simulink model "BSC"  (R2015b)
settings: Solver=FixedStepDiscrete  StartTime=0.0  StopTime=inf  FixedStep=bsck_stepSize  RelTol=1e-3
PreLoadFcn:
  | openecu_make_rtw_hook('model_load',   'BSC')
PostLoadFcn:
  | openecu_make_rtw_hook('model_loaded', 'BSC')
InitFcn:
  | openecu_make_rtw_hook('model_init',   'BSC')
undefined symbols (not defined in the file or in its folder): bscv_LowFaultType, bscv_MediumFaultType, bscv_SevereFaultType
libraries: simulink x4
settings Model: Creator=nctzv8  LastModifiedBy=nctzv8
settings ConfigSet: Description=OpenECU configuration set for code generation under RTW-EC.
settings SolverCC: PositivePriorityOrder=on
settings DataIOCC: SaveFormat=Array  SignalLoggingSaveFormat=ModelDataLogs
settings OptimizationCC: DefaultParameterBehavior=Inlined  InlineInvariantSignals=on  ExpressionDepthLimit=2147483647  StateBitsets=on  DataBitsets=on  ZeroExternalMemoryAtStartup=off  ZeroInternalMemoryAtStartup=off  NoFixptDivByZeroProtection=on  EfficientFloat2IntCast=on  OptimizeModelRefInitCode=on  LifeSpan=1
settings DebuggingCC: SaveWithParameterizedLinksMsg=none  UnderspecifiedInitializationDetection=Classic  MergeDetectMultiDrivingBlocksExec=none  SignalResolutionControl=TryResolveAllWithWarning  MultiTaskDSMMsg=warning  MultiTaskCondExecSysMsg=none  SingleTaskRateTransMsg=error  CheckMatrixSingularityMsg=warning  VectorMatrixConversionMsg=warning  FcnCallInpInsideContextMsg=UseLocalSettings  SignalLabelMismatchMsg=warning  StateNameClashWarn=warning
settings HardwareCC: ProdBitPerPointer=32  ProdLargestAtomicInteger=Long  ProdLargestAtomicFloat=Double  ProdEndianess=BigEndian  ProdWordSize=32  ProdHWDeviceType=Freescale->32-bit PowerPC  TargetIntDivRoundTo=Zero  TargetEndianess=BigEndian  TargetHWDeviceType=Freescale->32-bit PowerPC  ProdEqTarget=off
settings RTWCC: SystemTargetFile=openecu_ert.tlc  MakeCommand=make_rtw optimized_floating_point=1  TemplateMakefile=openecu_ert_r2015b_64.tmf  Description=OpenECU Platform Target (ERT, optimised floating-point code)  GenerateReport=on  RetainRTWFile=on  IncludeHyperlinkInReport=on  LaunchReport=on
settings CodeAppCC: ForceParamTrailComments=on  IgnoreCustomStorageClasses=off  SimulinkDataObjDesc=on  CustomSymbolStrType=$N$R$M  InsertBlockDesc=on  InternalIdentifier=Classic
settings STFCustomTargetCC: TargetLibSuffix=.a  GenerateSampleERTMain=on  ConcurrentExecutionCompliant=off  IncludeMdlTerminateFcn=off  GeneratePreprocessorConditionals=Use local settings  CombineOutputUpdateFcns=on  IncludeFileDelimiter=UseQuote  ERTCustomFileBanners=on  SupportContinuousTime=off  MATLABClassNameForMDSCustomization=Simulink.SoftwareTarget.ERTCustomization  CPPClassGenCompliant=off  GRTInterface=off  SystemTargetFile=openecu_ert.tlc
settings ERTTargetCC: GenerateSampleERTMain=on  ParMdlRefBuildCompliant=off  CompOptLevelCompliant=off  ConcurrentExecutionCompliant=off  IncludeMdlTerminateFcn=off  ERTFirstTimeCompliant=off  IncludeFileDelimiter=UseQuote  SupportNonInlinedSFcns=on  ModelStepFunctionPrototypeControlCompliant=off  CPPClassGenCompliant=off  UseToolchainInfoCompliant=off  ExtModeMexFile=noextcomm  InlinedParameterPlacement=NonHierarchical  ERTSrcFileBannerTemplate=oe_code_c_template.cgt  ERTHdrFileBannerTemplate=oe_code_h_template.cgt  ERTDataSrcFileTemplate=oe_data_c_template.cgt  ERTDataHdrFileTemplate=oe_data_h_template.cgt  ERTCustomFileTemplate=example_file_process.tlc  GlobalDataDefinition=InSeparateSourceFile  GlobalDataReference=InSeparateHeaderFile  EnableUserReplacementTypes=on

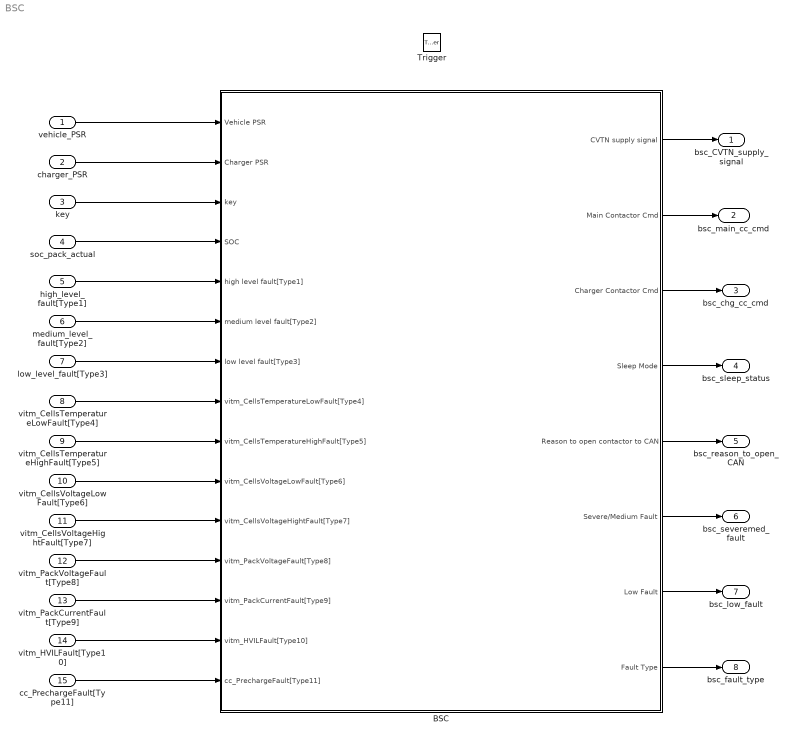
== system BSC ==
  vehicle_PSR : Inport  OutDataTypeStr=uint8  PortDimensions=1
  charger_PSR : Inport  Port=2  OutDataTypeStr=uint8  PortDimensions=1
  key : Inport  Port=3  OutDataTypeStr=uint8  PortDimensions=1
  soc_pack_actual : Inport  Port=4  OutDataTypeStr=double  PortDimensions=1
  high_level_fault[Type1] : Inport  Port=5  OutDataTypeStr=uint8  PortDimensions=1
  medium_level_fault[Type2] : Inport  Port=6  OutDataTypeStr=uint8  PortDimensions=1
  low_level_fault[Type3] : Inport  Port=7  OutDataTypeStr=uint8  PortDimensions=1
  vitm_CellsTemperatureLowFault[Type4] : Inport  Port=8  OutDataTypeStr=uint8  PortDimensions=1
  vitm_CellsTemperatureHighFault[Type5] : Inport  Port=9  OutDataTypeStr=uint8  PortDimensions=1
  vitm_CellsVoltageLowFault[Type6] : Inport  Port=10  OutDataTypeStr=uint8  PortDimensions=1
  vitm_CellsVoltageHightFault[Type7] : Inport  Port=11  OutDataTypeStr=uint8  PortDimensions=1
  vitm_PackVoltageFault[Type8] : Inport  Port=12  OutDataTypeStr=uint8  PortDimensions=1
  vitm_PackCurrentFault[Type9] : Inport  Port=13  OutDataTypeStr=uint8  PortDimensions=1
  vitm_HVILFault[Type10] : Inport  Port=14  OutDataTypeStr=uint8  PortDimensions=1
  cc_PrechargeFault[Type11] : Inport  Port=15  OutDataTypeStr=uint8  PortDimensions=1
  Trigger : TriggerPort  TriggerType=function-call  PortDimensions=1
  BSC : Subsystem  TreatAsAtomicUnit=on
  bsc_CVTN_supply_signal : Outport  OutDataTypeStr=boolean  PortDimensions=1
  bsc_main_cc_cmd : Outport  Port=2  OutDataTypeStr=boolean  PortDimensions=1
  bsc_chg_cc_cmd : Outport  Port=3  OutDataTypeStr=boolean  PortDimensions=1
  bsc_sleep_status : Outport  Port=4  OutDataTypeStr=boolean  PortDimensions=1
  bsc_reason_to_open_CAN : Outport  Port=5  OutDataTypeStr=uint8  PortDimensions=1
  bsc_severemed_fault : Outport  Port=6  OutDataTypeStr=uint8  PortDimensions=1
  bsc_low_fault : Outport  Port=7  OutDataTypeStr=uint8  PortDimensions=1
  bsc_fault_type : Outport  Port=8  OutDataTypeStr=uint8  PortDimensions=1
  wires:
  vehicle_PSR/1 -> BSC/1(Vehicle PSR)
  charger_PSR/1 -> BSC/2(Charger PSR)
  key/1 -> BSC/3(key)
  soc_pack_actual/1 -> BSC/4(SOC)
  high_level_fault[Type1]/1 -> BSC/5(high level fault[Type1])
  medium_level_fault[Type2]/1 -> BSC/6(medium level fault[Type2])
  low_level_fault[Type3]/1 -> BSC/7(low level fault[Type3])
  vitm_CellsTemperatureLowFault[Type4]/1 -> BSC/8(vitm_CellsTemperatureLowFault[Type4])
  vitm_CellsTemperatureHighFault[Type5]/1 -> BSC/9(vitm_CellsTemperatureHighFault[Type5])
  vitm_CellsVoltageLowFault[Type6]/1 -> BSC/10(vitm_CellsVoltageLowFault[Type6])
  vitm_CellsVoltageHightFault[Type7]/1 -> BSC/11(vitm_CellsVoltageHightFault[Type7])
  vitm_PackVoltageFault[Type8]/1 -> BSC/12(vitm_PackVoltageFault[Type8])
  vitm_PackCurrentFault[Type9]/1 -> BSC/13(vitm_PackCurrentFault[Type9])
  cc_PrechargeFault[Type11]/1 -> BSC/15(cc_PrechargeFault[Type11])
  BSC/1(CVTN supply signal) -> bsc_CVTN_supply_signal/1
  BSC/2(Main Contactor Cmd) -> bsc_main_cc_cmd/1
  BSC/3(Charger Contactor Cmd) -> bsc_chg_cc_cmd/1
  BSC/4(Sleep Mode) -> bsc_sleep_status/1
  BSC/5(Reason to open contactor to CAN) -> bsc_reason_to_open_CAN/1
  BSC/6(Severe/Medium Fault) -> bsc_severemed_fault/1
  BSC/7(Low Fault) -> bsc_low_fault/1
  BSC/8(Fault Type) -> bsc_fault_type/1
  vitm_HVILFault[Type10]/1 -> BSC/14(vitm_HVILFault[Type10])

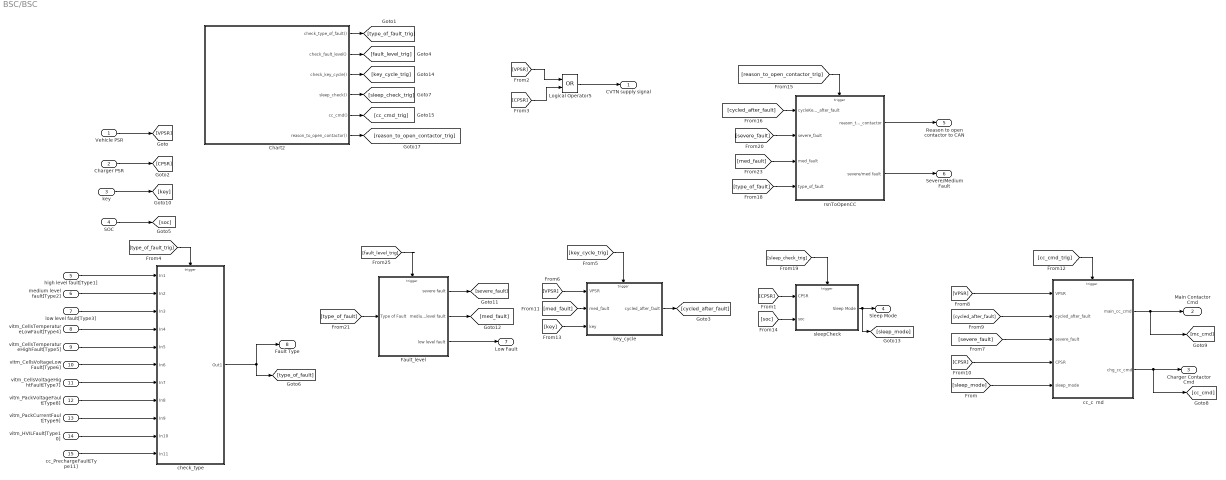
== system BSC/BSC ==
  Vehicle PSR : Inport  OutDataTypeStr=uint8  PortDimensions=1
  Charger PSR : Inport  Port=2  OutDataTypeStr=uint8  PortDimensions=1
  key : Inport  Port=3  OutDataTypeStr=uint8  PortDimensions=1
  SOC : Inport  Port=4  OutDataTypeStr=double  PortDimensions=1
  high level fault[Type1] : Inport  Port=5  OutDataTypeStr=uint8  PortDimensions=1
  medium level fault[Type2] : Inport  Port=6  OutDataTypeStr=uint8  PortDimensions=1
  low level fault[Type3] : Inport  Port=7  OutDataTypeStr=uint8  PortDimensions=1
  vitm_CellsTemperatureLowFault[Type4] : Inport  Port=8  OutDataTypeStr=uint8  PortDimensions=1
  vitm_CellsTemperatureHighFault[Type5] : Inport  Port=9  OutDataTypeStr=uint8  PortDimensions=1
  vitm_CellsVoltageLowFault[Type6] : Inport  Port=10  OutDataTypeStr=uint8  PortDimensions=1
  vitm_CellsVoltageHightFault[Type7] : Inport  Port=11  OutDataTypeStr=uint8  PortDimensions=1
  vitm_PackVoltageFault[Type8] : Inport  Port=12  OutDataTypeStr=uint8  PortDimensions=1
  vitm_PackCurrentFault[Type9] : Inport  Port=13  OutDataTypeStr=uint8  PortDimensions=1
  vitm_HVILFault[Type10] : Inport  Port=14  OutDataTypeStr=uint8  PortDimensions=1
  cc_PrechargeFault[Type11] : Inport  Port=15  OutDataTypeStr=uint8  PortDimensions=1
  Chart2 : Stateflow chart  TreatAsAtomicUnit=on
  Fault_level : Subsystem
  Logical Operator5 : Logic  Operator=OR  AllPortsSameDT=off  OutDataTypeStr=boolean
  cc_c  md : Subsystem
  check_type : Subsystem
  key_cycle : Subsystem
  rsnToOpenCC : Subsystem
  sleepCheck : Subsystem
  CVTN supply signal : Outport  OutDataTypeStr=boolean  PortDimensions=1
  Main Contactor Cmd : Outport  Port=2  OutDataTypeStr=boolean  PortDimensions=1
  Charger Contactor Cmd : Outport  Port=3  OutDataTypeStr=boolean  PortDimensions=1
  Sleep Mode : Outport  Port=4  OutDataTypeStr=boolean  PortDimensions=1
  Reason to open contactor to CAN : Outport  Port=5  OutDataTypeStr=uint8  PortDimensions=1
  Severe/Medium Fault : Outport  Port=6  OutDataTypeStr=uint8  PortDimensions=1
  Low Fault : Outport  Port=7  OutDataTypeStr=uint8  PortDimensions=1
  Fault Type : Outport  Port=8  OutDataTypeStr=uint8  PortDimensions=1
  wires:
  check_type/1(Out1) -> Fault Type/1, [type_of_fault]
  high level fault[Type1]/1 -> check_type/1(In1)
  vitm_CellsVoltageHightFault[Type7]/1 -> check_type/7(In7)
  vitm_PackVoltageFault[Type8]/1 -> check_type/8(In8)
  [key] -> key_cycle/3(key)
  vitm_CellsVoltageLowFault[Type6]/1 -> check_type/6(In6)
  [med_fault] -> key_cycle/2(med_fault)
  Charger PSR/1 -> [CPSR]
  key/1 -> [key]
  medium level fault[Type2]/1 -> check_type/2(In2)
  low level fault[Type3]/1 -> check_type/3(In3)
  vitm_CellsTemperatureHighFault[Type5]/1 -> check_type/5(In5)
  Logical Operator5/1 -> CVTN supply signal/1
  vitm_PackCurrentFault[Type9]/1 -> check_type/9(In9)
  key_cycle/1(cycled_after_fault) -> [cycled_after_fault]
  Vehicle PSR/1 -> [VPSR]
  Fault_level/1(severe fault) -> [severe_fault]
  Fault_level/3(low level fault) -> Low Fault/1
  [VPSR] -> key_cycle/1(VPSR)
  vitm_CellsTemperatureLowFault[Type4]/1 -> check_type/4(In4)
  [VPSR] -> Logical Operator5/1
  Fault_level/2(medium level fault) -> [med_fault]
  [type_of_fault] -> Fault_level/1(Type of Fault)
  [CPSR] -> Logical Operator5/2
  SOC/1 -> [soc]
  [fault_level_trig] -> Fault_level/Trigger
  Chart2/3(check_key_cycle()) -> [key_cycle_trig]
  [cc_cmd_trig] -> cc_c  md/Trigger
  [sleep_mode] -> cc_c  md/5(sleep_mode)
  [severe_fault] -> cc_c  md/3(severe_fault)
  rsnToOpenCC/2(severe/med fault) -> Severe/Medium Fault/1
  [cycled_after_fault] -> cc_c  md/2(cycled_after_fault)
  [med_fault] -> rsnToOpenCC/3(med_fault)
  Chart2/2(check_fault_level()) -> [fault_level_trig]
  Chart2/5(cc_cmd()) -> [cc_cmd_trig]
  [CPSR] -> cc_c  md/4(CPSR)
  Chart2/6(reason_to_open_contactor()) -> [reason_to_open_contactor_trig]
  [type_of_fault_trig] -> check_type/Trigger
  [key_cycle_trig] -> key_cycle/Trigger
  cc_c  md/2(chg_cc_cmd) -> Charger Contactor Cmd/1, [cc_cmd]
  rsnToOpenCC/1(reason_to_open_contactor) -> Reason to open contactor to CAN/1
  [reason_to_open_contactor_trig] -> rsnToOpenCC/Trigger
  [VPSR] -> cc_c  md/1(VPSR)
  [severe_fault] -> rsnToOpenCC/2(severe_fault)
  [type_of_fault] -> rsnToOpenCC/4(type_of_fault)
  cc_c  md/1(main_cc_cmd) -> Main Contactor Cmd/1, [mc_cmd]
  Chart2/1(check_type_of_fault()) -> [type_of_fault_trig]
  Chart2/4(sleep_check()) -> [sleep_check_trig]
  [CPSR] -> sleepCheck/1(CPSR)
  [soc] -> sleepCheck/2(soc)
  sleepCheck/1(Sleep Mode) -> [sleep_mode], Sleep Mode/1
  [sleep_check_trig] -> sleepCheck/Trigger
  [cycled_after_fault] -> rsnToOpenCC/1(cycleKey_after_fault)
  cc_PrechargeFault[Type11]/1 -> check_type/11(In11)
  vitm_HVILFault[Type10]/1 -> check_type/10(In10)

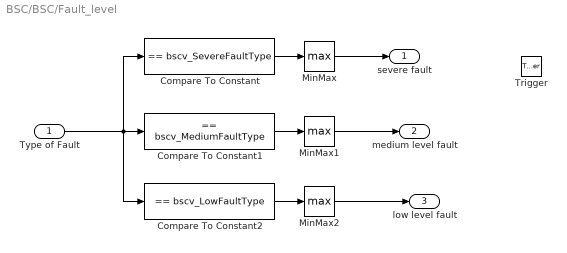
== system BSC/BSC/Fault_level ==
  Type of Fault : Inport
  Trigger : TriggerPort  TriggerType=function-call  PortDimensions=1
  Compare To Constant : simulink/Logic and Bit Operations/Compare To Constant  relop===  const=bscv_SevereFaultType  OutDataTypeStr=uint8
  Compare To Constant1 : simulink/Logic and Bit Operations/Compare To Constant  relop===  const=bscv_MediumFaultType  OutDataTypeStr=uint8
  Compare To Constant2 : simulink/Logic and Bit Operations/Compare To Constant  relop===  const=bscv_LowFaultType  OutDataTypeStr=uint8
  MinMax : MinMax  Function=max
  MinMax1 : MinMax  Function=max
  MinMax2 : MinMax  Function=max
  severe fault : Outport
  medium level fault : Outport  Port=2
  low level fault : Outport  Port=3
  wires:
  MinMax/1 -> severe fault/1
  MinMax1/1 -> medium level fault/1
  MinMax2/1 -> low level fault/1
  Compare To Constant1/1 -> MinMax1/1
  Type of Fault/1 -> Compare To Constant1/1, Compare To Constant2/1, Compare To Constant/1
  Compare To Constant2/1 -> MinMax2/1
  Compare To Constant/1 -> MinMax/1

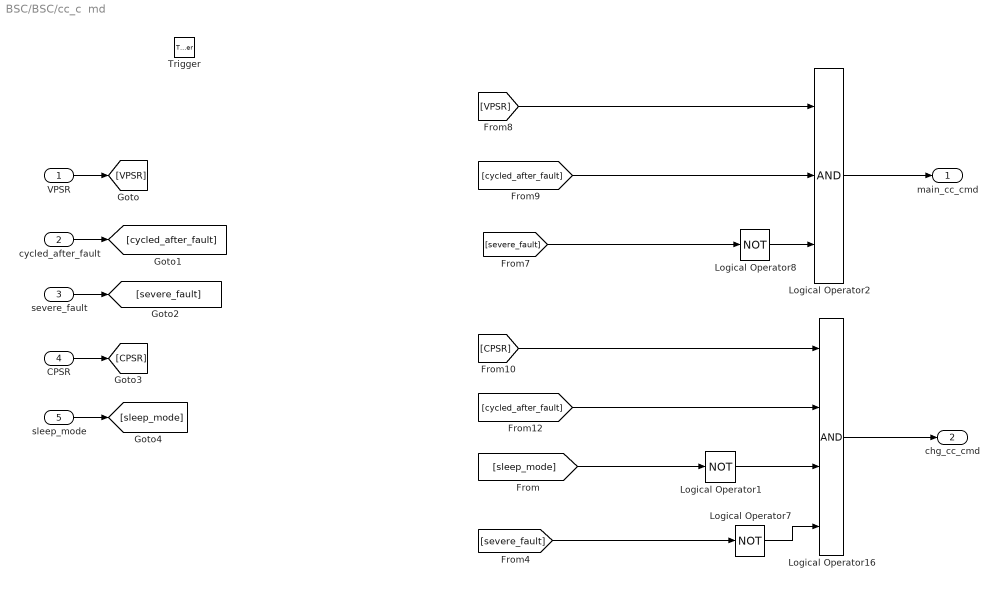
== system BSC/BSC/cc_c  md ==
  VPSR : Inport
  cycled_after_fault : Inport  Port=2
  severe_fault : Inport  Port=3
  CPSR : Inport  Port=4
  sleep_mode : Inport  Port=5
  Trigger : TriggerPort  TriggerType=function-call  PortDimensions=1
  Logical Operator1 : Logic  Operator=NOT  Inputs=1  AllPortsSameDT=off  OutDataTypeStr=boolean
  Logical Operator16 : Logic  Inputs=4  AllPortsSameDT=off  OutDataTypeStr=boolean
  Logical Operator2 : Logic  Inputs=3  AllPortsSameDT=off  OutDataTypeStr=boolean
  Logical Operator7 : Logic  Operator=NOT  Inputs=1  AllPortsSameDT=off  OutDataTypeStr=boolean
  Logical Operator8 : Logic  Operator=NOT  Inputs=1  AllPortsSameDT=off  OutDataTypeStr=boolean
  main_cc_cmd : Outport
  chg_cc_cmd : Outport  Port=2
  wires:
  [sleep_mode] -> Logical Operator1/1
  Logical Operator8/1 -> Logical Operator2/3
  Logical Operator7/1 -> Logical Operator16/4
  Logical Operator1/1 -> Logical Operator16/3
  Logical Operator16/1 -> chg_cc_cmd/1
  Logical Operator2/1 -> main_cc_cmd/1
  [VPSR] -> Logical Operator2/1
  [cycled_after_fault] -> Logical Operator2/2
  [severe_fault] -> Logical Operator8/1
  [CPSR] -> Logical Operator16/1
  [cycled_after_fault] -> Logical Operator16/2
  [severe_fault] -> Logical Operator7/1
  VPSR/1 -> [VPSR]
  cycled_after_fault/1 -> [cycled_after_fault]
  severe_fault/1 -> [severe_fault]
  CPSR/1 -> [CPSR]
  sleep_mode/1 -> [sleep_mode]

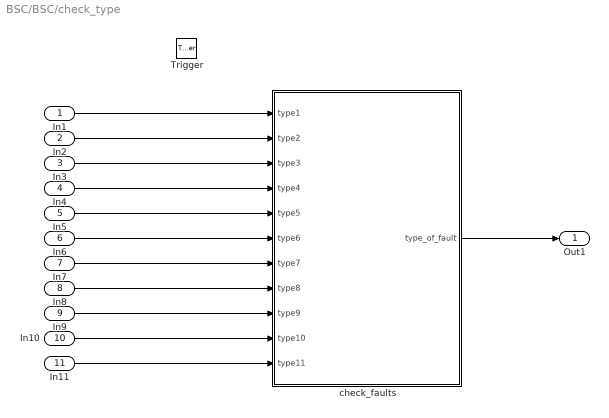
== system BSC/BSC/check_type ==
  In1 : Inport
  In2 : Inport  Port=2
  In3 : Inport  Port=3
  In4 : Inport  Port=4
  In5 : Inport  Port=5
  In6 : Inport  Port=6
  In7 : Inport  Port=7
  In8 : Inport  Port=8
  In9 : Inport  Port=9
  In10 : Inport  Port=10
  In11 : Inport  Port=11
  Trigger : TriggerPort  TriggerType=function-call  PortDimensions=1
  check_faults : Stateflow chart  TreatAsAtomicUnit=on
  Out1 : Outport
  wires:
  check_faults/1(type_of_fault) -> Out1/1
  In8/1 -> check_faults/8(type8)
  In2/1 -> check_faults/2(type2)
  In4/1 -> check_faults/4(type4)
  In6/1 -> check_faults/6(type6)
  In7/1 -> check_faults/7(type7)
  In5/1 -> check_faults/5(type5)
  In3/1 -> check_faults/3(type3)
  In9/1 -> check_faults/9(type9)
  In1/1 -> check_faults/1(type1)
  In10/1 -> check_faults/10(type10)
  In11/1 -> check_faults/11(type11)

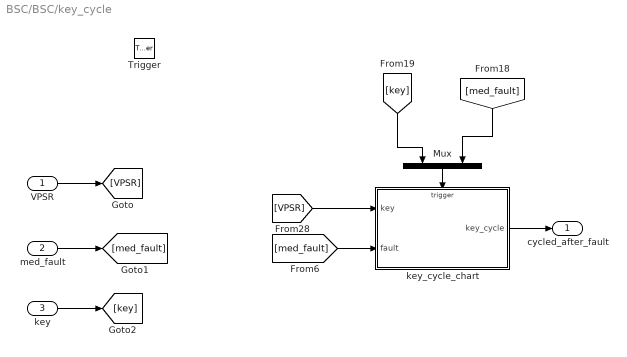
== system BSC/BSC/key_cycle ==
  VPSR : Inport
  med_fault : Inport  Port=2
  key : Inport  Port=3
  Trigger : TriggerPort  TriggerType=function-call  PortDimensions=1
  Mux : Mux  Inputs=2
  key_cycle_chart : Stateflow chart  TreatAsAtomicUnit=on
  cycled_after_fault : Outport
  wires:
  Mux/1 -> key_cycle_chart/Trigger
  [key] -> Mux/1
  key_cycle_chart/1(key_cycle) -> cycled_after_fault/1
  [VPSR] -> key_cycle_chart/1(key)
  [med_fault] -> key_cycle_chart/2(fault)
  [med_fault] -> Mux/2
  VPSR/1 -> [VPSR]
  med_fault/1 -> [med_fault]
  key/1 -> [key]

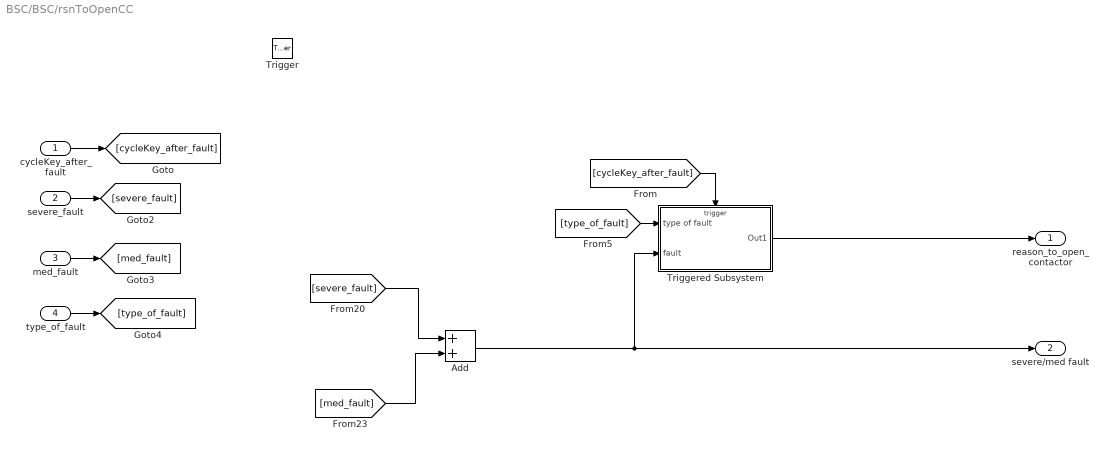
== system BSC/BSC/rsnToOpenCC ==
  cycleKey_after_fault : Inport
  severe_fault : Inport  Port=2
  med_fault : Inport  Port=3
  type_of_fault : Inport  Port=4
  Trigger : TriggerPort  TriggerType=function-call  PortDimensions=1
  Add : Sum  AccumDataTypeStr=uint8  OutDataTypeStr=uint8  InputSameDT=on
  Triggered Subsystem : Subsystem  TreatAsAtomicUnit=on
  reason_to_open_contactor : Outport
  severe/med fault : Outport  Port=2
  wires:
  [type_of_fault] -> Triggered Subsystem/1(type of fault)
  Triggered Subsystem/1(Out1) -> reason_to_open_contactor/1
  [severe_fault] -> Add/1
  [med_fault] -> Add/2
  Add/1 -> severe/med fault/1, Triggered Subsystem/2(fault)
  cycleKey_after_fault/1 -> [cycleKey_after_fault]
  severe_fault/1 -> [severe_fault]
  med_fault/1 -> [med_fault]
  type_of_fault/1 -> [type_of_fault]
  [cycleKey_after_fault] -> Triggered Subsystem/Trigger

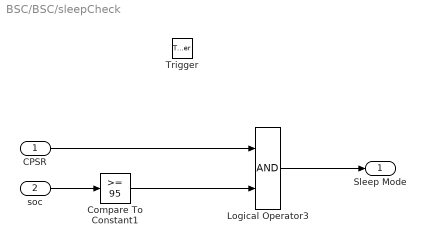
== system BSC/BSC/sleepCheck ==
  CPSR : Inport
  soc : Inport  Port=2
  Trigger : TriggerPort  TriggerType=function-call  PortDimensions=1
  Compare To Constant1 : simulink/Logic and Bit Operations/Compare To Constant  relop=>=  const=95  OutDataTypeStr=boolean
  Logical Operator3 : Logic  AllPortsSameDT=off  OutDataTypeStr=boolean
  Sleep Mode : Outport  OutDataTypeStr=boolean  PortDimensions=1
  wires:
  CPSR/1 -> Logical Operator3/1
  soc/1 -> Compare To Constant1/1
  Compare To Constant1/1 -> Logical Operator3/2
  Logical Operator3/1 -> Sleep Mode/1

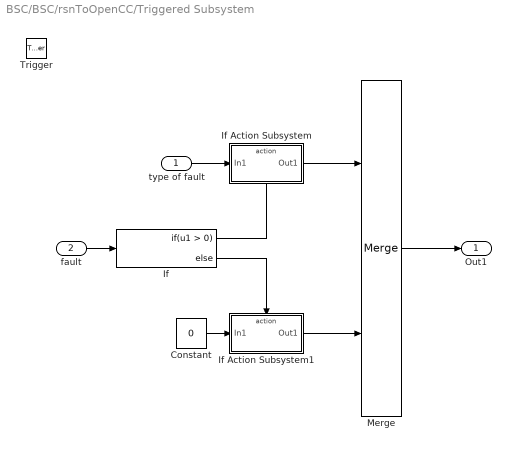
== system BSC/BSC/rsnToOpenCC/Triggered Subsystem ==
  type of fault : Inport
  fault : Inport  Port=2
  Trigger : TriggerPort  TriggerType=either
  Constant : Constant  Value=0  OutDataTypeStr=uint8
  If : If
  If Action Subsystem : Subsystem  TreatAsAtomicUnit=on
  If Action Subsystem1 : Subsystem  TreatAsAtomicUnit=on
  Merge : Merge
  Out1 : Outport
  wires:
  fault/1 -> If/1
  type of fault/1 -> If Action Subsystem/1(In1)
  Constant/1 -> If Action Subsystem1/1(In1)
  Merge/1 -> Out1/1
  If Action Subsystem1/1(Out1) -> Merge/2
  If Action Subsystem/1(Out1) -> Merge/1
  If/2 -> If Action Subsystem1/Action
  If/1 -> If Action Subsystem/Action

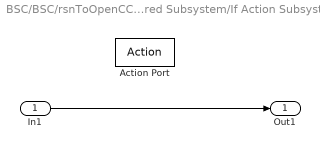
== system BSC/BSC/rsnToOpenCC/Triggered Subsystem/If Action Subsystem ==
  In1 : Inport
  Action Port : ActionPort  ActionType=then
  Out1 : Outport
  wires:
  In1/1 -> Out1/1

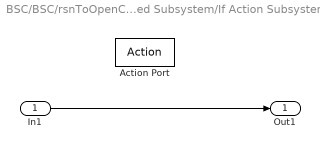
== system BSC/BSC/rsnToOpenCC/Triggered Subsystem/If Action Subsystem1 ==
  In1 : Inport
  Action Port : ActionPort  ActionType=else
  Out1 : Outport
  wires:
  In1/1 -> Out1/1

== stateflow chart BSC/key_cycle/key_cycle_chart ==
  state inital_key_off_fault
    entry:
    key_cycle = 0;
    off_fault = 1;
  state Key_OFF
    entry:
    key_state = OFF;
    exit:
    on_fault = 0 ;
    (default) -> (junction 84)
    (junction 84) -> (junction 86) [order 1] : key_change [on_fault==0]
    (junction 84) -> (junction 87) [order 2]
    (junction 86) -> (junction 83) : {off_store = off_store+1;}
    (junction 83) -> (junction 87)
    (junction 87) -> (junction 73)
    (junction 73) -> (junction 74) [order 1] : [off_store>1]
    (junction 73) -> (junction 75) [order 2]
    (junction 74) -> (junction 76) : {off_store=1;}
    (junction 76) -> (junction 75)
    (junction 75) -> (junction 77)
    (junction 77) -> (junction 40)
    (junction 40) -> (junction 41) [order 1] : [fault==1]
    (junction 40) -> (junction 94) [order 2]
    (junction 41) -> (junction 43) : {key_cycle = 0;
        | off_store=0;
        | on_store=0;
        | off_fault = 1 ;}
    (junction 94) -> (junction 90) [order 1] : [off_store==1]
    (junction 94) -> (junction 89) [order 2]
    (junction 90) -> (junction 95) : {key_cycle = 1;}
    (junction 95) -> (junction 89)
    (junction 89) -> (junction 42)
    (junction 43) -> (junction 42)
    (junction 42) -> (junction 44)
  state Key_ON
    entry:
    key_state = ON
    exit:
    off_fault = 0 ;
    (default) -> (junction 121)
    (junction 121) -> (junction 113) [order 1] : key_change [off_fault==0]
    (junction 121) -> (junction 112) [order 2]
    (junction 113) -> (junction 122) : {on_store = on_store+1;}
    (junction 122) -> (junction 112)
    (junction 112) -> (junction 135)
    (junction 135) -> (junction 137) [order 1] : [on_store>1]
    (junction 135) -> (junction 138) [order 2]
    (junction 137) -> (junction 134) : {on_store=1;}
    (junction 134) -> (junction 138)
    (junction 138) -> (junction 136)
    (junction 136) -> (junction 107)
    (junction 107) -> (junction 104) [order 1] : [fault==1]
    (junction 107) -> (junction 118) [order 2]
    (junction 104) -> (junction 101) : {key_cycle = 0;
        | on_store=0;
        | off_store=0;
        | on_fault = 1 ;}
    (junction 118) -> (junction 116) [order 1] : [on_store==1]
    (junction 118) -> (junction 128) [order 2]
    (junction 116) -> (junction 127) : {key_cycle = 1;}
    (junction 127) -> (junction 128)
    (junction 128) -> (junction 109)
    (junction 101) -> (junction 109)
    (junction 109) -> (junction 106)
  (default) -> inital_key_off_fault [order 2]
  (default) -> Key_ON [order 1] : key_change
  Key_OFF -> Key_OFF [order 2] : fault_change
  Key_ON -> Key_ON [order 2] : fault_change
  inital_key_off_fault -> Key_ON : key_change
  Key_OFF -> Key_ON [order 1] : key_change
  Key_ON -> Key_OFF [order 1] : key_change
  data: key input; key_cycle output uint8 =1; key_state local uint8 =0; OFF constant uint8 size=1 =0; ON constant uint8 size=1 =1; fault input; cycle_state local uint8 =0; off_store local uint8 =0; on_store local uint8 =0; off_fault local uint8 =0; on_fault local uint8 =0
  events: key_change input EITHER_EDGE_EVENT; fault_change input EITHER_EDGE_EVENT

== stateflow chart BSC/Chart2 ==
  state main
    (default) -> (junction 3)
    main -> (junction 3)
    (junction 3) -> (junction 18) : {check_type_of_fault;}
    (junction 18) -> (junction 11) : {check_fault_level;}
    (junction 11) -> (junction 22) : {check_key_cycle;}
    (junction 22) -> (junction 1) : {sleep_check;}
    (junction 1) -> (junction 13) : {cc_cmd;}
    (junction 13) -> (junction 9) : {reason_to_open_contactor;}
  events: check_type_of_fault output FUNCTION_CALL_EVENT; check_fault_level output FUNCTION_CALL_EVENT; check_key_cycle output FUNCTION_CALL_EVENT; sleep_check output FUNCTION_CALL_EVENT; cc_cmd output FUNCTION_CALL_EVENT; reason_to_open_contactor output FUNCTION_CALL_EVENT

== stateflow chart BSC/check_type/check_faults ==
  (default) -> (junction 88)
  (junction 89) -> (junction 145) : {type_of_fault = 1;}
  (junction 88) -> (junction 89) [order 1] : [type1]
  (junction 88) -> (junction 90) [order 2]
  (junction 145) -> (junction 144)
  (junction 91) -> (junction 144) : {type_of_fault = 2;}
  (junction 90) -> (junction 91) [order 1] : [type2]
  (junction 90) -> (junction 92) [order 2]
  (junction 144) -> (junction 143)
  (junction 93) -> (junction 143) : {type_of_fault = 3;}
  (junction 92) -> (junction 93) [order 1] : [type3]
  (junction 92) -> (junction 102) [order 2]
  (junction 143) -> (junction 159)
  (junction 102) -> (junction 103) [order 1] : [type4]
  (junction 103) -> (junction 159) : {type_of_fault = 4;}
  (junction 102) -> (junction 107) [order 2]
  (junction 159) -> (junction 161)
  (junction 107) -> (junction 104) [order 1] : [type5]
  (junction 104) -> (junction 161) : {type_of_fault = 5;}
  (junction 107) -> (junction 112) [order 2]
  (junction 161) -> (junction 152)
  (junction 112) -> (junction 110) [order 1] : [type6]
  (junction 110) -> (junction 152) : {type_of_fault = 6;}
  (junction 112) -> (junction 115) [order 2]
  (junction 152) -> (junction 154)
  (junction 115) -> (junction 113) [order 1] : [type7]
  (junction 113) -> (junction 154) : {type_of_fault = 7;}
  (junction 115) -> (junction 117) [order 2]
  (junction 154) -> (junction 147)
  (junction 117) -> (junction 116) [order 1] : [type8]
  (junction 116) -> (junction 147) : {type_of_fault = 8;}
  (junction 117) -> (junction 120) [order 2]
  (junction 147) -> (junction 149)
  (junction 119) -> (junction 149) : {type_of_fault = 9;}
  (junction 120) -> (junction 119) [order 1] : [type9]
  (junction 120) -> (junction 173) [order 2]
  (junction 149) -> (junction 172)
  (junction 171) -> (junction 172) : {type_of_fault = 10;}
  (junction 173) -> (junction 171) [order 1] : [type10]
  (junction 173) -> (junction 182) [order 2]
  (junction 172) -> (junction 183)
  (junction 184) -> (junction 183) : {type_of_fault = 11;}
  (junction 182) -> (junction 184) [order 1] : [type11]
  (junction 182) -> (junction 162) [order 2]
  (junction 183) -> (junction 164)
  (junction 162) -> (junction 164) : {type_of_fault = 0;}
  (junction 164) -> (junction 167)
  data: type1 input uint8; type2 input uint8; type3 input uint8; type4 input uint8; type5 input uint8; type_of_fault output uint8; type6 input uint8; type7 input uint8; type8 input uint8; type9 input uint8; type10 input uint8; type11 input uint8
